simulink model "soc_pmsm_singlecpu_ref"  (R2023b)
settings: Solver=FixedStepAuto  StartTime=0.0  StopTime=1  RelTol=1e-3  EnableMultiTasking=on
InitFcn:
  | soc_mcb_pmsm_foc_sensorless_f28379d_data;
  | coeff = .007*Ts/50e-6;
model workspace (MAT data in the model file):
  mwTaskManagerKernelLatency = 0
values from neighbouring files (symbols this model uses):
  dataType = 'single'    [soc_mcb_pmsm_foc_sensorless_f28379d_data.m]
  inverter = mcb_SetInverterParameters('BoostXL-DRV8305')    [soc_mcb_pmsm_foc_sensorless_f28379d_data.m]
  PI_params = mcb.internal.SetControllerParameters(pmsm,inverter,PU_System,T_pwm,2*Ts,Ts_speed)    [soc_mcb_pmsm_foc_sensorless_f28379d_data.m]
  pmsm = mcb_SetPMSMMotorParameters('custom')    [soc_mcb_pmsm_foc_sensorless_f28379d_data.m]
  PU_System = mcb_SetPUSystem(pmsm,inverter)    [soc_mcb_pmsm_foc_sensorless_f28379d_data.m]
  Ts = T_pwm    (= 5e-05)    [soc_mcb_pmsm_foc_sensorless_f28379d_data.m]
  Ts_speed = 10*Ts    (= 0.0005)    [soc_mcb_pmsm_foc_sensorless_f28379d_data.m]
  Vd_Ref_openLoop_PU = Speed_openLoop_PU    (= 0.1)    [soc_mcb_pmsm_foc_sensorless_f28379d_data.m]
undefined symbols (not defined in the file or in its folder): soc_pmsm_singlecpu_ref
libraries: mcbcontrolslib x10, prociolib x5, simulink x4, slpidlib x3, mcbpositiondecoderlib x2
settings Model: ExtModeTrigDuration=8  Creator=The MathWorks, Inc.  LastModifiedBy=The MathWorks, Inc.
settings SolverCC: AlgebraicLoopSolver=TrustRegion  PositivePriorityOrder=on  MaxZcPerStep=1
settings DataIOCC: SaveOutput=off  DSMLogging=off
settings OptimizationCC: DefaultUnderspecifiedDataType=single  EnhancedBackFolding=on  PassReuseOutputArgsAs=Individual arguments  MaxStackSize=1024  OptimizeBlockOrder=speed  DifferentSizesBufferReuse=on  OptimizationCustomize=off  DenormalBehavior=FlushToZero  EfficientTunableParamExpr=on
settings DebuggingCC: IntegerOverflowMsg=none  ParameterPrecisionLossMsg=none  ParameterTunabilityLossMsg=error  UnconnectedInputMsg=warning  UnconnectedOutputMsg=warning  UnconnectedLineMsg=warning
settings HardwareCC: ProdBitPerChar=16  ProdBitPerInt=16  ProdBitPerPointer=32  ProdBitPerSizeT=32  ProdBitPerPtrDiffT=32  ProdLargestAtomicInteger=Integer  ProdLargestAtomicFloat=None  ProdWordSize=16  ProdLongLongMode=on  ProdHWDeviceType=Texas Instruments->C2000  HardwareBoardFeatureSet=SoCBlockset
settings ModelReferenceCC: EnableRefExpFcnMdlSchedulingChecks=on  ModelReferenceNumInstancesAllowed=Single
settings SFSimCC: MATLABDynamicMemAlloc=off
settings RTWCC: Description=Embedded Coder  SystemTargetFile=ert.tlc  HardwareBoard=TI Delfino F28379D LaunchPad  TLCOptions="-aInlineSetEventsForThisBaseRateFcn=TLC_FALSE -aSuppressMultiTaskScheduler=TLC_FALSE   -aRateBasedStepFcn=1"  TemplateMakefile=ert_default_tmf  Toolchain=Texas Instruments Code Composer Studio (C2000)  DLArmComputeVersion=19.05
settings CodeAppCC: ForceParamTrailComments=on  IgnoreCustomStorageClasses=off  MaxIdLength=64  OperatorAnnotations=on  SimulinkDataObjDesc=on  SFDataObjDesc=on  InsertBlockDesc=on
settings ERTTargetCC: CodeReplacementLibrary=TI C28x  ExtModeTransport=4  ExtModeStaticAlloc=on  ExtModeStaticAllocSize=10000  ExtModeMexFile=ext_xcp  ExtModeIntrfLevel=Level2 - Open

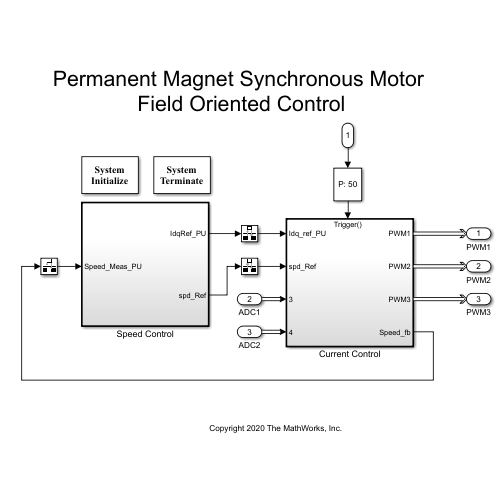
[thumbnail: Simulink's stored preview of the top-level diagram]
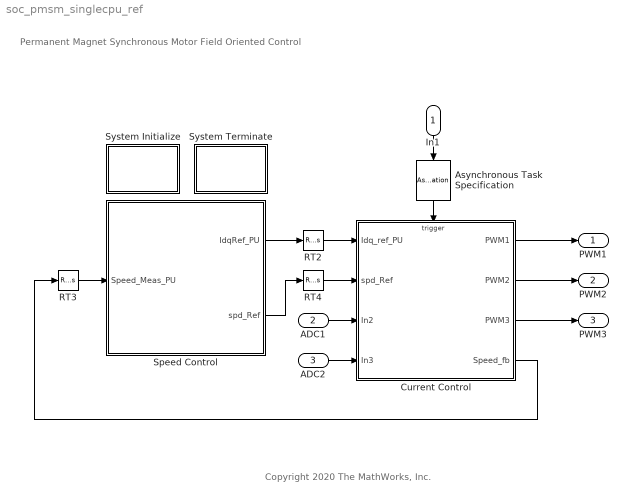
== system soc_pmsm_singlecpu_ref ==
  note: Permanent Magnet Synchronous Motor
      | Field Oriented Control
  note: Copyright 2020 The MathWorks, Inc.
  In1 : Inport  OutputFunctionCall=on
  ADC1 : Inport  OutputPortMessageModes=m  Port=2
  ADC2 : Inport  OutputPortMessageModes=m  Port=3
  Asynchronous Task Specification : AsynchronousTaskSpecification  TaskPriority=50
  Current Control : Subsystem
  RT2 : RateTransition  Deterministic=off
  RT3 : RateTransition  Deterministic=off  OutPortSampleTime=Ts_speed
  RT4 : RateTransition  Deterministic=off
  Speed Control : Subsystem  TreatAsAtomicUnit=on  SystemSampleTime=Ts_speed
  System Initialize : Subsystem  mask(System Initialize){ShowInLibBrowser=0}
      mask prompts: ShowInLibBrowser "Simulink:masks:CustCodeMaskParam1_MP"
      settings: CopyFcn=cccopyfcn(gcb)  OpenFcn=ccopenfcn('System Initialize Function')
      mask Help: eval('feval(''rtwprivate'',''rtwhelpview'',''rtw_sys_initialize_block'')');
      mask Display: disp('System\nInitialize');
  System Terminate : Subsystem  mask(System Terminate){ShowInLibBrowser=0}
      mask prompts: ShowInLibBrowser "Simulink:masks:CustCodeMaskParam1_MP"
      settings: CopyFcn=cccopyfcn(gcb)  OpenFcn=ccopenfcn('System Terminate Function')
      mask Help: eval('feval(''rtwprivate'',''rtwhelpview'',''rtw_sys_terminate_block'')');
      mask Display: disp('System\nTerminate');
  PWM1 : Outport  InputPortMessageModes=m
  PWM2 : Outport  InputPortMessageModes=m  Port=2
  PWM3 : Outport  InputPortMessageModes=m  Port=3
  wires:
  RT2/1 -> Current Control/1(Idq_ref_PU)
  ADC2/1 -> Current Control/4(In3)
  Current Control/4(Speed_fb) -> RT3/1
  ADC1/1 -> Current Control/3(In2)
  In1/1 -> Asynchronous Task Specification/1
  Current Control/2(PWM2) -> PWM2/1
  Current Control/1(PWM1) -> PWM1/1
  Current Control/3(PWM3) -> PWM3/1
  Speed Control/1(IdqRef_PU) -> RT2/1
  RT3/1 -> Speed Control/1(Speed_Meas_PU)
  RT4/1 -> Current Control/2(spd_Ref)
  Asynchronous Task Specification/1 -> Current Control/Trigger
  Speed Control/2(spd_Ref) -> RT4/1

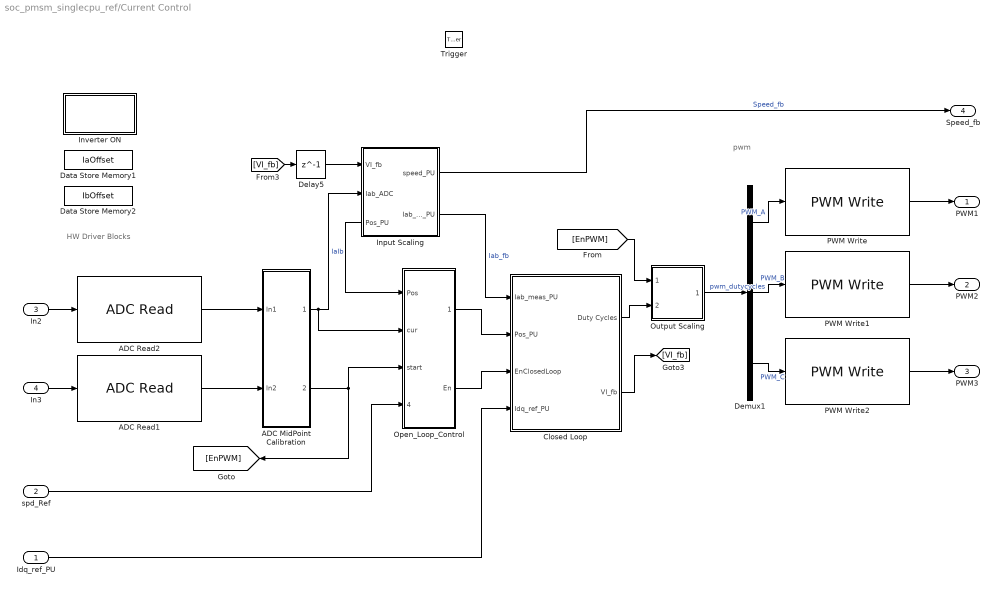
== system soc_pmsm_singlecpu_ref/Current Control ==
  note: pwm
  note: HW Driver Blocks
  Idq_ref_PU : Inport
  spd_Ref : Inport  Port=2
  In2 : Inport  Port=3
  In3 : Inport  Port=4
  Trigger : TriggerPort  TriggerType=function-call  VariantControl=Variant  PortDimensions=1
  ADC MidPoint Calibration : Subsystem
  ADC Read1 : prociolib/ADC Read  DataType=uint16  SampleTime=-1  NumCh=1  PeripheralConfigBtnCtrl=0  BlockSID=soc_pmsm_singlecpu_ref:512
  ADC Read2 : prociolib/ADC Read  DataType=uint16  SampleTime=-1  NumCh=1  PeripheralConfigBtnCtrl=0  BlockSID=soc_pmsm_singlecpu_ref:717
  Closed Loop : Subsystem
  Data Store Memory1 : DataStoreMemory  DataStoreName=IaOffset  ReadBeforeWriteMsg=warning  WriteAfterWriteMsg=warning  WriteAfterReadMsg=warning  InitialValue=inverter.CtSensAOffset  ShowAdditionalParam=off
  Data Store Memory2 : DataStoreMemory  DataStoreName=IbOffset  ReadBeforeWriteMsg=warning  WriteAfterWriteMsg=warning  WriteAfterReadMsg=warning  InitialValue=inverter.CtSensBOffset  ShowAdditionalParam=off
  Delay5 : Delay  DelayLength=1
  Demux1 : Demux  Outputs=3
  Input Scaling : Subsystem
      settings: PortSchema="{\"entries\":[{\"content\":{\"sides\":[{\"content\":{\"connectorIds\":[\"In1\",\"In2\",\"Out3\"]},\"type\":\"ConnectorPlacement.EquallySpacedRectSide\",\"uuid\":\"6d6167e7-0996-4b81-a35a-1346d5f5bdac\"},{\"content\":{\"connectorIds\":[\"Out1\",\"Out2\"],\"side\":\"RIGHT\"},\"type\":\"ConnectorPlacement.EquallySpacedRectSide\",\"uuid\":\"bac86f6f-215c-4b7d-8f06-4a6da7918799\"},{\"content\":{\"connectorIds\":[],\"side\":\"TOP\"},\"type\":\"ConnectorPlacement.EquallySpacedRectSide\",\"uuid\":\"65876525-48d1-40c6-98ca-4ecaae4f0bb2\"},{\"content\":{\"connectorIds\":[],\"side\":\"HIDDEN\"},\"type\":\"ConnectorPlacement.EquallySpacedRectSide\",\"uuid\":\"fe89acd2-2a3e-478b-951b-0712bf130e60\"}]},\"type\":\"ConnectorPlacement.EquallySpacedConnector\",\"uuid\":\"d7bb3362-92d6-4e3b-9b7c-91cd383782b7\"}],\"packageUris\":[\"http://schema.mathworks.com/mf0/Connector/R2020b\"],\"version\":\"1.0\"}"
  Inverter ON : Subsystem  mask(System Outputs){ShowInLibBrowser=0}
      mask prompts: ShowInLibBrowser "Simulink:masks:CustCodeMaskParam1_MP"
      settings: CopyFcn=cccopyfcn(gcb)  OpenFcn=ccopenfcn('System Outputs Function')
      mask Help: eval('feval(''rtwprivate'',''rtwhelpview'',''rtw_sys_outputs_block'')');
      mask Display: disp('System\nOutputs');
  Open_Loop_Control : Subsystem
  Output Scaling : Subsystem
  PWM Write : prociolib/PWM Write  ShowPeriodInp=off  ShowPhaseInp=off  PeripheralConfigBtnCtrl=0  BlockSID=soc_pmsm_singlecpu_ref:666
  PWM Write1 : prociolib/PWM Write  ShowPeriodInp=off  ShowPhaseInp=off  PeripheralConfigBtnCtrl=0  BlockSID=soc_pmsm_singlecpu_ref:667
  PWM Write2 : prociolib/PWM Write  ShowPeriodInp=off  ShowPhaseInp=off  PeripheralConfigBtnCtrl=0  BlockSID=soc_pmsm_singlecpu_ref:668
  PWM1 : Outport
  PWM2 : Outport  Port=2
  PWM3 : Outport  Port=3
  Speed_fb : Outport  Port=4  InitialOutput=0  VectorParamsAs1DForOutWhenUnconnected=off
  wires:
  Closed Loop/1(Duty Cycles) -> Output Scaling/2(Vabc_ref)
  Delay5/1 -> Input Scaling/1(VI_fb)
  Output Scaling/1(PWM_Duty_Cycles) -> Demux1/1  "pwm_dutycycles"
  Closed Loop/2(VI_fb) -> [VI_fb]
  PWM Write1/1 -> PWM2/1
  In3/1 -> ADC Read1/1
  Input Scaling/2(Iab_meas_PU) -> Closed Loop/1(Iab_meas_PU)  "Iab_fb"
  Input Scaling/1(speed_PU) -> Speed_fb/1  "Speed_fb"
  In2/1 -> ADC Read2/1
  [VI_fb] -> Delay5/1
  ADC Read2/1 -> ADC MidPoint Calibration/1(In1)
  Idq_ref_PU/1 -> Closed Loop/4(Idq_ref_PU)
  ADC Read1/1 -> ADC MidPoint Calibration/2(In2)
  PWM Write2/1 -> PWM3/1
  PWM Write/1 -> PWM1/1
  Demux1/3 -> PWM Write2/1  "PWM_C"
  Demux1/2 -> PWM Write1/1  "PWM_B"
  Demux1/1 -> PWM Write/1  "PWM_A"
  ADC MidPoint Calibration/1(Iab_ADC) -> Open_Loop_Control/2(cur), Input Scaling/2(Iab_ADC)  "IaIb"
  spd_Ref/1 -> Open_Loop_Control/4(spd_Ref)
  Open_Loop_Control/1(Pos_PU) -> Closed Loop/2(Pos_PU)
  Open_Loop_Control/2(En) -> Closed Loop/3(EnClosedLoop)
  ADC MidPoint Calibration/2(EnPWM) -> [EnPWM], Open_Loop_Control/3(start)
  [EnPWM] -> Output Scaling/1(EnPWM)
  Input Scaling/3(Pos_PU) -> Open_Loop_Control/1(Pos)

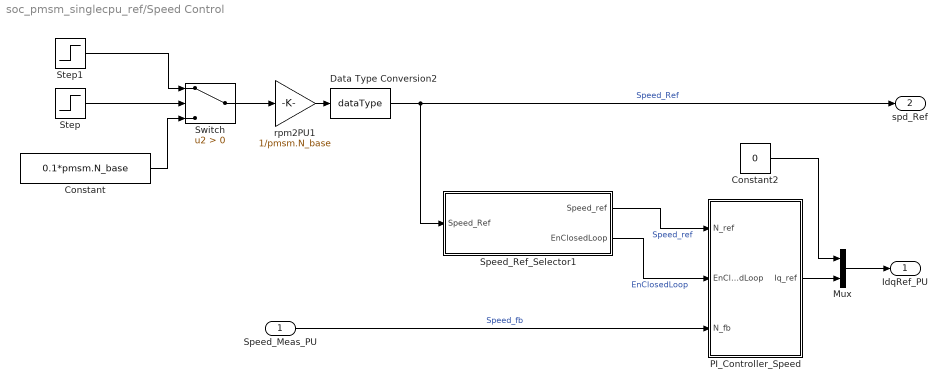
== system soc_pmsm_singlecpu_ref/Speed Control ==
  Speed_Meas_PU : Inport
  Constant : Constant  Value=0.1*pmsm.N_base  SampleTime=-1
  Constant2 : Constant  Value=0  OutDataTypeStr=dataType
  Data Type Conversion2 : DataTypeConversion  OutDataTypeStr=dataType  RndMeth=Simplest  SaturateOnIntegerOverflow=off
  Mux : Mux  Inputs=2
  PI_Controller_Speed : Subsystem
  Speed_Ref_Selector1 : Subsystem
  Step : Step  Time=.05
  Step1 : Step  Time=.3  Before=0.5*pmsm.N_base  After=0.7*pmsm.N_base
  Switch : Switch  Criteria=u2 > Threshold  SaturateOnIntegerOverflow=off  InputSameDT=off
  rpm2PU1 : Gain  Gain=1/pmsm.N_base  RndMeth=Simplest  OutDataTypeStr=Inherit: Same as input
  IdqRef_PU : Outport  VectorParamsAs1DForOutWhenUnconnected=off
  spd_Ref : Outport  Port=2  VectorParamsAs1DForOutWhenUnconnected=off
  wires:
  Speed_Meas_PU/1 -> PI_Controller_Speed/3(N_fb)  "Speed_fb"
  Mux/1 -> IdqRef_PU/1
  Constant2/1 -> Mux/1
  PI_Controller_Speed/1(Iq_ref) -> Mux/2
  Data Type Conversion2/1 -> Speed_Ref_Selector1/1(Speed_Ref), spd_Ref/1  "Speed_Ref"
  rpm2PU1/1 -> Data Type Conversion2/1
  Speed_Ref_Selector1/1(Speed_ref) -> PI_Controller_Speed/1(N_ref)  "Speed_ref"
  Speed_Ref_Selector1/2(EnClosedLoop) -> PI_Controller_Speed/2(EnClosedLoop)  "EnClosedLoop"
  Constant/1 -> Switch/3
  Step/1 -> Switch/2
  Step1/1 -> Switch/1
  Switch/1 -> rpm2PU1/1

== system soc_pmsm_singlecpu_ref/System Initialize ==

== system soc_pmsm_singlecpu_ref/System Terminate ==

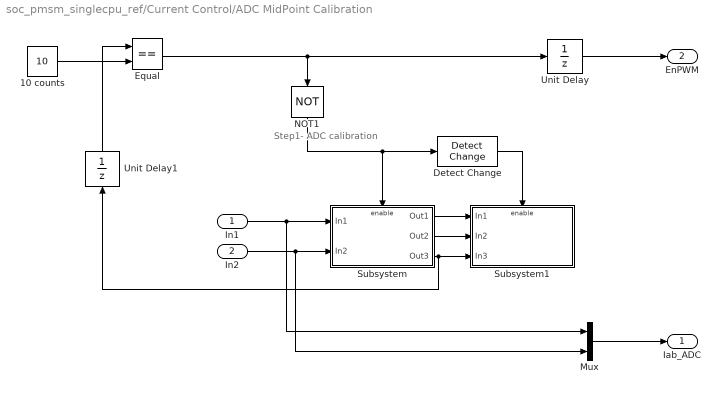
== system soc_pmsm_singlecpu_ref/Current Control/ADC MidPoint Calibration ==
  note: Step1- ADC calibration
  In1 : Inport
  In2 : Inport  Port=2
  10 counts : Constant  Value=10
  Detect Change : simulink/Logic and Bit Operations/Detect Change  vinit=1  OutDataTypeStr=boolean
  Equal : RelationalOperator  Operator===  OutDataTypeStr=boolean  RndMeth=Simplest  InputSameDT=off
  Mux : Mux  Inputs=2
  NOT1 : Logic  Operator=NOT  IconShape=distinctive  AllPortsSameDT=off  OutDataTypeStr=boolean
  Subsystem : Subsystem
  Subsystem1 : Subsystem
  Unit Delay : UnitDelay  SampleTime=-1  HasFrameUpgradeWarning=on
  Unit Delay1 : UnitDelay  SampleTime=-1  HasFrameUpgradeWarning=on
  Iab_ADC : Outport
  EnPWM : Outport  Port=2
  wires:
  Equal/1 -> NOT1/1, Unit Delay/1
  Subsystem/1(Out1) -> Subsystem1/1(In1)
  Detect Change/1 -> Subsystem1/Enable
  Subsystem/3(Out3) -> Unit Delay1/1, Subsystem1/3(In3)
  Subsystem/2(Out2) -> Subsystem1/2(In2)
  In1/1 -> Mux/1, Subsystem/1(In1)
  In2/1 -> Mux/2, Subsystem/2(In2)
  Mux/1 -> Iab_ADC/1
  Unit Delay/1 -> EnPWM/1
  NOT1/1 -> Subsystem/Enable, Detect Change/1
  Unit Delay1/1 -> Equal/1
  10 counts/1 -> Equal/2

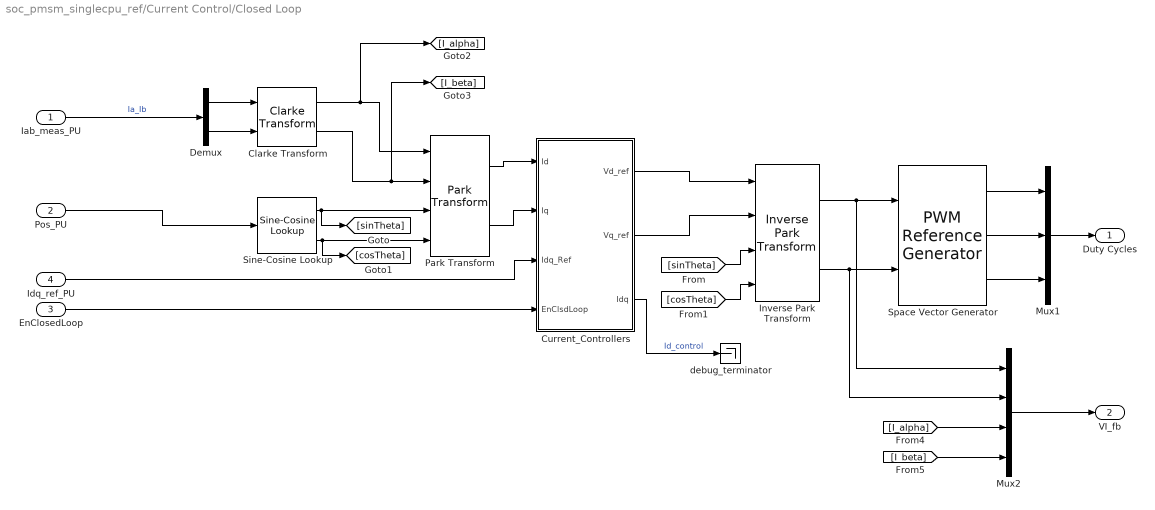
== system soc_pmsm_singlecpu_ref/Current Control/Closed Loop ==
  Iab_meas_PU : Inport
  Pos_PU : Inport  Port=2
  EnClosedLoop : Inport  Port=3
  Idq_ref_PU : Inport  Port=4
  Clarke Transform : mcbcontrolslib/Clarke Transform  VariantControl=Variant2  PhaseInput=Two inputs  EnPowerInv=off
  Current_Controllers : Subsystem
  Demux : Demux  Outputs=2
  Inverse Park Transform : mcbcontrolslib/Inverse Park Transform  PhaseInput=Two inputs  AxisAlignment=D-axis  ThetaInput=Sine and Cosine electrical position  AngleInput=Per-unit  N_points=1024
  Mux1 : Mux  Inputs=3
  Mux2 : Mux
  Park Transform : mcbcontrolslib/Park Transform  PhaseInput=Two inputs  AxisAlignment=D-axis  ThetaInput=Sine and Cosine electrical position  AngleInput=Per-unit  N_points=1024
  Sine-Cosine Lookup : mcbcontrolslib/Sine-Cosine Lookup  AngleInput=Per-unit  N_points=1024
  Space Vector Generator : mcbcontrolslib/PWM Reference Generator  inSignal=Valphabeta  modType=SVM: space vector modulation
  debug_terminator : Terminator
  Duty Cycles : Outport  VectorParamsAs1DForOutWhenUnconnected=off
  VI_fb : Outport  Port=2  VectorParamsAs1DForOutWhenUnconnected=off
  wires:
  Current_Controllers/1(Vd_ref) -> Inverse Park Transform/1
  [cosTheta] -> Inverse Park Transform/4
  [I_beta] -> Mux2/4
  Inverse Park Transform/2 -> Space Vector Generator/2, Mux2/2
  Inverse Park Transform/1 -> Space Vector Generator/1, Mux2/1
  [sinTheta] -> Inverse Park Transform/3
  Mux2/1 -> VI_fb/1
  Clarke Transform/1 -> [I_alpha], Park Transform/1
  Current_Controllers/2(Vq_ref) -> Inverse Park Transform/2
  Clarke Transform/2 -> [I_beta], Park Transform/2
  Sine-Cosine Lookup/1 -> [sinTheta], Park Transform/3
  [I_alpha] -> Mux2/3
  Space Vector Generator/1 -> Mux1/1
  Space Vector Generator/3 -> Mux1/3
  Mux1/1 -> Duty Cycles/1
  Sine-Cosine Lookup/2 -> Park Transform/4, [cosTheta]
  Space Vector Generator/2 -> Mux1/2
  Park Transform/1 -> Current_Controllers/1(Id)
  Park Transform/2 -> Current_Controllers/2(Iq)
  Demux/1 -> Clarke Transform/1
  Demux/2 -> Clarke Transform/2
  Iab_meas_PU/1 -> Demux/1  "Ia_Ib"
  Idq_ref_PU/1 -> Current_Controllers/3(Idq_Ref)
  Current_Controllers/3(Idq) -> debug_terminator/1  "Id_control"
  Pos_PU/1 -> Sine-Cosine Lookup/1
  EnClosedLoop/1 -> Current_Controllers/4(EnClsdLoop)

== system soc_pmsm_singlecpu_ref/Current Control/Input Scaling ==
  note: This filter is required to correct DC offset,
      | which helps to estimate position more accurately.
  note: Current Measurements
  note: Position & Speed Measurements
  VI_fb : Inport
  Iab_ADC : Inport  Port=2
  Calculate Phase Currents : Subsystem
  Calculate position and speed : Subsystem
  High pass filter : Subsystem
  speed_PU : Outport
  Iab_meas_PU : Outport  Port=2
  Pos_PU : Outport  Port=3
  wires:
  Calculate Phase Currents/1(Iab_meas_PU) -> Iab_meas_PU/1
  Iab_ADC/1 -> Calculate Phase Currents/1(Iab_ADC)
  VI_fb/1 -> High pass filter/1(In1)
  Calculate position and speed/2(Pos_PU) -> Pos_PU/1
  Calculate position and speed/1(speed_PU) -> speed_PU/1
  High pass filter/1(Out1) -> Calculate position and speed/1(VI_fb)

== system soc_pmsm_singlecpu_ref/Current Control/Inverter ON ==

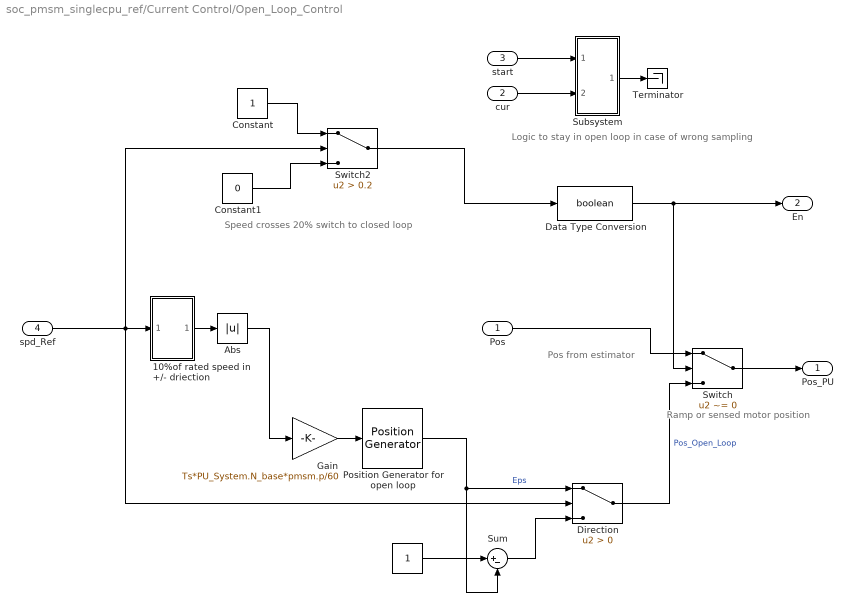
== system soc_pmsm_singlecpu_ref/Current Control/Open_Loop_Control ==
  note: Logic to stay in open loop in case of wrong sampling
  note: Speed crosses 20% switch to closed loop
  note: Pos from estimator
  note: Ramp or sensed motor position
  Pos : Inport
  cur : Inport  Port=2
  start : Inport  Port=3
  spd_Ref : Inport  Port=4
  " " : Constant  OutDataTypeStr=dataType  SampleTime=-1
  10%of rated speed in +/- driection : Subsystem
  Abs : Abs  SaturateOnIntegerOverflow=off
  Constant : Constant  OutDataTypeStr=uint16
  Constant1 : Constant  Value=0  OutDataTypeStr=uint16
  Data Type Conversion : DataTypeConversion  OutDataTypeStr=boolean  RndMeth=Simplest  SaturateOnIntegerOverflow=off
  Direction : Switch  Criteria=u2 > Threshold  OutDataTypeStr=dataType  RndMeth=Simplest  SaturateOnIntegerOverflow=off  InputSameDT=off
  Gain : Gain  Gain=Ts*PU_System.N_base*pmsm.p/60  OutDataTypeStr=Inherit: Same as input  ParamDataTypeStr=Inherit: Same as input
  Position Generator for open loop : mcbcontrolslib/Position Generator  AngleOutput=Per-unit  ExternalReset=none  Offset=0
  Subsystem : Subsystem
  Sum : Sum  Inputs=|+-  RndMeth=Simplest  OutDataTypeStr=Inherit: Same as first input
  Switch : Switch  Criteria=u2 ~= 0  Threshold=0.1  SaturateOnIntegerOverflow=off  InputSameDT=off
  Switch2 : Switch  Criteria=u2 > Threshold  Threshold=0.2  SaturateOnIntegerOverflow=off  InputSameDT=off
  Terminator : Terminator
  Pos_PU : Outport
  En : Outport  Port=2
  wires:
  Constant1/1 -> Switch2/3
  Constant/1 -> Switch2/1
  Pos/1 -> Switch/1
  Switch/1 -> Pos_PU/1
  Gain/1 -> Position Generator for open loop/1
  Switch2/1 -> Data Type Conversion/1
  spd_Ref/1 -> Switch2/2, Direction/2, 10%of rated speed in +/- driection/1(In1)
  Sum/1 -> Direction/3
  " "/1 -> Sum/1
  Position Generator for open loop/1 -> Direction/1, Sum/2  "Eps"
  Direction/1 -> Switch/3  "Pos_Open_Loop"
  Abs/1 -> Gain/1
  10%of rated speed in +/- driection/1(Out1) -> Abs/1
  cur/1 -> Subsystem/2(In1)
  start/1 -> Subsystem/1(start)
  Data Type Conversion/1 -> En/1, Switch/2
  Subsystem/1(Close) -> Terminator/1

== system soc_pmsm_singlecpu_ref/Current Control/Output Scaling ==
  EnPWM : Inport
  Vabc_ref : Inport  Port=2
  Constant : Constant  Value=0.5  OutDataTypeStr=dataType  SampleTime=-1
  Constant1 : Constant  Value=0  OutDataTypeStr=single
  Mux : Mux  Inputs=3
  One_by_Two : Gain  Gain=0.5  RndMeth=Simplest  OutDataTypeStr=Inherit: Same as input
  Sum : Sum  Inputs=|++
  Switch : Switch  Criteria=u2 > Threshold  SaturateOnIntegerOverflow=off  InputSameDT=off
  PWM_Duty_Cycles : Outport
  wires:
  Constant/1 -> Sum/2
  Vabc_ref/1 -> One_by_Two/1
  One_by_Two/1 -> Sum/1
  Mux/1 -> Switch/3
  Constant1/1 -> Mux/3, Mux/1, Mux/2
  Sum/1 -> Switch/1  "PWM_Duty_Cycles"
  EnPWM/1 -> Switch/2
  Switch/1 -> PWM_Duty_Cycles/1  "pwm_dutycycles"

== system soc_pmsm_singlecpu_ref/Speed Control/PI_Controller_Speed ==
  N_ref : Inport
  EnClosedLoop : Inport  Port=2
  N_fb : Inport  Port=3
  Discrete PI Controller with anti-windup & reset : slpidlib/PID Controller  Controller=PI  Form=Parallel  TimeDomain=Discrete-time  UseExternalTs=off  SampleTime=-1  IntegratorMethod=Forward Euler  FilterMethod=Forward Euler  ControllerParametersSource=external  P=1  I=1  UseKiTs=on  D=0  N=100  UseFilter=on  TunerSelectOption=Transfer Function Based (PID Tuner App)  InitialConditionSource=external  InitialConditionForIntegrator=0  InitialConditionForFilter=0  DifferentiatorICPrevScaledInput=0  ExternalReset=level  TrackingMode=off  Kt=1  LimitOutput=on  SatLimitsSource=internal  UpperSaturationLimit=1  LowerSaturationLimit=-1  LinearizeAsGain=on  AntiWindupMode=clamping  Kb=1  LimitIntegrator=off  UpperIntegratorSaturationLimit=inf  LowerIntegratorSaturationLimit=-inf  RndMeth=Simplest  POutMin=[]  POutMax=[]  IOutMin=[]  IOutMax=[]  DOutMin=[]  DOutMax=[]  NOutMin=[]  NOutMax=[]  SumOutMin=[]  SumOutMax=[]  SaturationOutDataTypeStr=Inherit: Inherit via back propagation  SaturationOutMin=[]  SaturationOutMax=[]  PParamMin=[]  PParamMax=[]  IParamMin=[]  IParamMax=[]  DParamMin=[]  DParamMax=[]  NParamMin=[]  NParamMax=[]  KbParamMin=[]  KbParamMax=[]  KtParamMin=[]  KtParamMax=[]  KbOutMin=[]  KbOutMax=[]  KtOutMin=[]  KtOutMax=[]  IntegratorOutMin=[]  IntegratorOutMax=[]  FilterOutMin=[]  FilterOutMax=[]  SumI1OutMin=[]  SumI1OutMax=[]  SumI2OutMin=[]  SumI2OutMax=[]  SumI3OutMin=[]  SumI3OutMax=[]  SumI4OutMin=[]  SumI4OutMax=[]  SumDOutMin=[]  SumDOutMax=[]  DifferentiatorOutMin=[]  DifferentiatorOutMax=[]  FilterDiffOutCoefMin=[]  FilterDiffOutCoefMax=[]  ReciprocalOutMin=[]  ReciprocalOutMax=[]  SumDenOutMin=[]  SumDenOutMax=[]  SumNumOutMin=[]  SumNumOutMax=[]  DivideOutMin=[]  DivideOutMax=[]  UdiffTsProdOutMin=[]  UdiffTsProdOutMax=[]  NTsProdOutMin=[]  NTsProdOutMax=[]  UintegralTsProdOutMin=[]  UintegralTsProdOutMax=[]  UngainTsProdOutMin=[]  UngainTsProdOutMax=[]  ClampingZeroOutDataTypeStr=Inherit: Inherit via back propagation  ClampingZeroOutMin=[]  ClampingZeroOutMax=[]  FilterDenConstantOutDataTypeStr=Inherit: Inherit via back propagation  FilterDenConstantOutMin=[]  FilterDenConstantOutMax=[]  PCopyOutDataTypeStr=Inherit: Inherit via back propagation  PCopyOutMin=[]  PCopyOutMax=[]  NCopyOutDataTypeStr=Inherit: Inherit via back propagation  NCopyOutMin=[]  NCopyOutMax=[]  IntegratorContinuousStateAttributes=''  IntegratorStateMustResolveToSignalObject=off  IntegratorRTWStateStorageClass=Auto  FilterContinuousStateAttributes=''  FilterStateMustResolveToSignalObject=off  FilterRTWStateStorageClass=Auto  ParallelPVariant=ExternalParameters  IdealPVariant=Disabled  IVariant=ExternalParameters  DVariant=Disabled  IntegratorVariant=Discrete  SatVariant=Enabled  AWVariant=DiscClampingParallel  PCopyVariant=Disabled  TRVariant=Disabled  FdbkBlocksVariant=Forward  IdealPFdbkVariant=Disabled  SatFdbkVariant=Disabled  DerivativeFilterVariant=Disabled  NVariant=Disabled  NCopyVariant=Disabled_SignalSpec  FilterICVariant=Disabled  IntegratorICVariant=ExternalICs  ExternalResetVariant=ExternalReset  TRSumVariant=Passthrough  SumFdbkVariant=Disabled  SumVariant=Sum_PI  TsampFilterVariant=InternalTs  TsampNgainVariant=Passthrough  TsampIntegralVariant=Disabled_SignalSpec  ExternalSaturationOutDataTypeStr=Inherit: Same as second input
      settings: LibrarySourceBlock=mcbcontrolslib/PI Controller
  Ki1 : Constant  Value=PI_params.Ki_speed*Ts_speed  OutDataTypeStr=dataType  SampleTime=-1
  Ki2 : Constant  Value=0  OutDataTypeStr=dataType  SampleTime=-1
  Kp1 : Constant  Value=PI_params.Kp_speed  OutDataTypeStr=dataType  SampleTime=-1
  Logical Operator : Logic  Operator=NOT  IconShape=distinctive  AllPortsSameDT=off  OutDataTypeStr=boolean
  Sum : Sum  Inputs=|+-  OutDataTypeStr=Inherit: Same as first input
  Iq_ref : Outport  VectorParamsAs1DForOutWhenUnconnected=off
  wires:
  Discrete PI Controller with anti-windup & reset/1 -> Iq_ref/1
  Ki1/1 -> Discrete PI Controller with anti-windup & reset/3
  Kp1/1 -> Discrete PI Controller with anti-windup & reset/2
  N_fb/1 -> Sum/2
  N_ref/1 -> Sum/1
  Sum/1 -> Discrete PI Controller with anti-windup & reset/1
  Logical Operator/1 -> Discrete PI Controller with anti-windup & reset/4
  Ki2/1 -> Discrete PI Controller with anti-windup & reset/5
  EnClosedLoop/1 -> Logical Operator/1

== system soc_pmsm_singlecpu_ref/Speed Control/Speed_Ref_Selector1 ==
  note: En Closed loop
  Speed_Ref : Inport
  Ki3 : Constant  Value=0  OutDataTypeStr=dataType  SampleTime=-1
  Ki4 : Constant  OutDataTypeStr=dataType  SampleTime=-1
  Switch2 : Switch  Criteria=u2 > Threshold  Threshold=.2  SaturateOnIntegerOverflow=off  InputSameDT=off
  Unit Delay : UnitDelay  SampleTime=-1  HasFrameUpgradeWarning=on
  Zero_Cancellation : mcbcontrolslib/IIR Filter  VariantControl=Low Pass Filter  VariantSelect=Low-pass  Filter_constant=.01*(Ts_speed/Ts)  advancedSettings=off  Ts=50e-6  cutOff_freq=1
  Speed_ref : Outport
  EnClosedLoop : Outport  Port=2
  wires:
  Speed_Ref/1 -> Unit Delay/1, Zero_Cancellation/1
  Switch2/1 -> EnClosedLoop/1
  Ki3/1 -> Switch2/3
  Ki4/1 -> Switch2/1
  Unit Delay/1 -> Switch2/2
  Zero_Cancellation/1 -> Speed_ref/1

== system soc_pmsm_singlecpu_ref/Current Control/ADC MidPoint Calibration/Subsystem ==
  In1 : Inport
  In2 : Inport  Port=2
  Enable : EnablePort
  Counter Free-Running : simulink/Sources/Counter Free-Running  NumBits=16  tsamp=-1
  Memory : Memory  InheritSampleTime=on
  Memory1 : Memory  InheritSampleTime=on
  Sum : Sum
  Sum1 : Sum
  Out1 : Outport  InitialOutput=2048
  Out2 : Outport  Port=2  InitialOutput=2048
  Out3 : Outport  Port=3  InitialOutput=2048
  wires:
  In1/1 -> Sum/1
  Memory/1 -> Sum/2
  Memory1/1 -> Sum1/2
  Sum/1 -> Memory/1, Out1/1
  In2/1 -> Sum1/1
  Sum1/1 -> Memory1/1, Out2/1
  Counter Free-Running/1 -> Out3/1

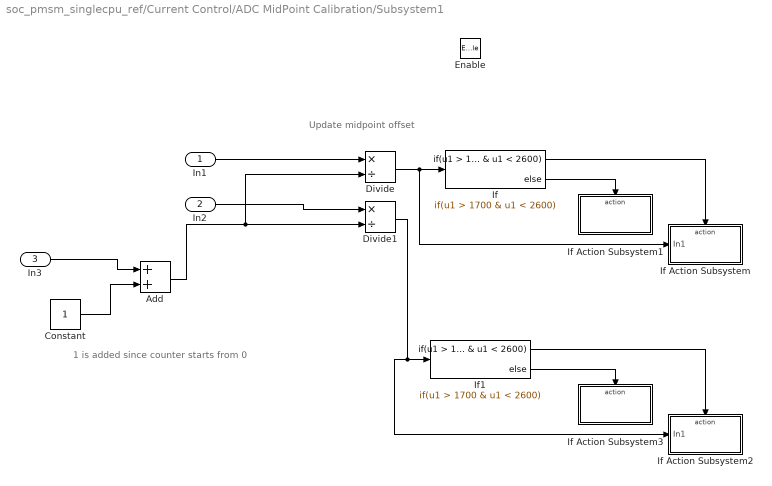
== system soc_pmsm_singlecpu_ref/Current Control/ADC MidPoint Calibration/Subsystem1 ==
  note: 1 is added since counter starts from 0
  note: Update midpoint offset
  In1 : Inport
  In2 : Inport  Port=2
  In3 : Inport  Port=3
  Enable : EnablePort
  Add : Sum
  Constant : Constant  SampleTime=-1
  Divide : Product  Inputs=*/  OutDataTypeStr=uint16
  Divide1 : Product  Inputs=*/  OutDataTypeStr=uint16
  If : If  IfExpression=u1 > 1700 & u1 < 2600
  If Action Subsystem : Subsystem  TreatAsAtomicUnit=on
  If Action Subsystem1 : Subsystem  TreatAsAtomicUnit=on
  If Action Subsystem2 : Subsystem  TreatAsAtomicUnit=on
  If Action Subsystem3 : Subsystem  TreatAsAtomicUnit=on
  If1 : If  IfExpression=u1 > 1700 & u1 < 2600
  wires:
  In1/1 -> Divide/1
  If1/2 -> If Action Subsystem3/Action
  In2/1 -> Divide1/1
  If1/1 -> If Action Subsystem2/Action
  Divide1/1 -> If Action Subsystem2/1(In1), If1/1
  If/1 -> If Action Subsystem/Action
  Add/1 -> Divide/2, Divide1/2
  If/2 -> If Action Subsystem1/Action
  Divide/1 -> If Action Subsystem/1(In1), If/1
  In3/1 -> Add/1
  Constant/1 -> Add/2

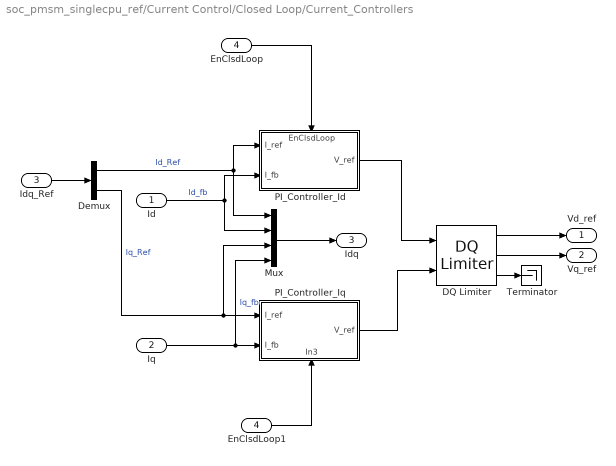
== system soc_pmsm_singlecpu_ref/Current Control/Closed Loop/Current_Controllers ==
  Id : Inport
  Iq : Inport  Port=2
  Idq_Ref : Inport  Port=3
  EnClsdLoop : Inport  Port=4
  DQ Limiter : mcbcontrolslib/DQ Limiter  satMethodInputType=Specify via dialog  satMethodSelected=D-Q equivalence  satLimitInputType=Specify via dialog  Vmax=0.95
  Demux : Demux  Outputs=2
  EnClsdLoop1 : InportShadow  Port=4
  Mux : Mux
  PI_Controller_Id : Subsystem
      settings: PortSchema="{\"entries\":[{\"content\":{\"sides\":[{\"content\":{\"connectorIds\":[\"In1\",\"In2\"]},\"type\":\"ConnectorPlacement.EquallySpacedRectSide\",\"uuid\":\"1dbe4538-5262-4de9-8cd0-6fe9721117d9\"},{\"content\":{\"connectorIds\":[\"Out1\"],\"side\":\"RIGHT\"},\"type\":\"ConnectorPlacement.EquallySpacedRectSide\",\"uuid\":\"73929c6b-82a2-4171-bcf4-852047833ed6\"},{\"content\":{\"connectorIds\":[\"In3\"],\"side\":\"TOP\"},\"type\":\"ConnectorPlacement.EquallySpacedRectSide\",\"uuid\":\"d145dc66-6457-4965-9d28-ee054dd23661\"},{\"content\":{\"connectorIds\":[],\"side\":\"HIDDEN\"},\"type\":\"ConnectorPlacement.EquallySpacedRectSide\",\"uuid\":\"26db549f-462f-46ef-aaa7-ab739cada5d6\"}]},\"type\":\"ConnectorPlacement.EquallySpacedConnector\",\"uuid\":\"507f0757-a119-4143-8cba-4226e39989e3\"}],\"packageUris\":[\"http://schema.mathworks.com/mf0/Connector/R2020b\"],\"version\":\"1.0\"}"
  PI_Controller_Iq : Subsystem
      settings: PortSchema="{\"entries\":[{\"content\":{\"sides\":[{\"content\":{\"connectorIds\":[\"In1\",\"In2\"]},\"type\":\"ConnectorPlacement.EquallySpacedRectSide\",\"uuid\":\"1dbe4538-5262-4de9-8cd0-6fe9721117d9\"},{\"content\":{\"connectorIds\":[\"Out1\"],\"side\":\"RIGHT\"},\"type\":\"ConnectorPlacement.EquallySpacedRectSide\",\"uuid\":\"73929c6b-82a2-4171-bcf4-852047833ed6\"},{\"content\":{\"connectorIds\":[],\"side\":\"TOP\"},\"type\":\"ConnectorPlacement.EquallySpacedRectSide\",\"uuid\":\"d145dc66-6457-4965-9d28-ee054dd23661\"},{\"content\":{\"connectorIds\":[\"In3\"],\"side\":\"BOTTOM\"},\"type\":\"ConnectorPlacement.EquallySpacedRectSide\",\"uuid\":\"758abaee-43c6-4dc5-aebc-88543f7390b7\"},{\"content\":{\"connectorIds\":[],\"side\":\"HIDDEN\"},\"type\":\"ConnectorPlacement.EquallySpacedRectSide\",\"uuid\":\"26db549f-462f-46ef-aaa7-ab739cada5d6\"}]},\"type\":\"ConnectorPlacement.EquallySpacedConnector\",\"uuid\":\"507f0757-a119-4143-8cba-4226e39989e3\"}],\"packageUris\":[\"http://schema.mathworks.com/mf0/Connector/R2020b\"],\"version\":\"1.0\"}"
  Terminator : Terminator
  Vd_ref : Outport  VectorParamsAs1DForOutWhenUnconnected=off
  Vq_ref : Outport  Port=2  VectorParamsAs1DForOutWhenUnconnected=off
  Idq : Outport  Port=3  VectorParamsAs1DForOutWhenUnconnected=off
  wires:
  Iq/1 -> Mux/4, PI_Controller_Iq/2(I_fb)  "Iq_fb"
  PI_Controller_Id/1(V_ref) -> DQ Limiter/1
  Id/1 -> PI_Controller_Id/2(I_fb), Mux/2  "Id_fb"
  Demux/1 -> PI_Controller_Id/1(I_ref), Mux/1  "Id_Ref"
  Demux/2 -> Mux/3, PI_Controller_Iq/1(I_ref)  "Iq_Ref"
  DQ Limiter/1 -> Vd_ref/1
  DQ Limiter/2 -> Vq_ref/1
  PI_Controller_Iq/1(V_ref) -> DQ Limiter/2
  DQ Limiter/3 -> Terminator/1
  Idq_Ref/1 -> Demux/1
  Mux/1 -> Idq/1
  EnClsdLoop/1 -> PI_Controller_Id/3(EnClsdLoop)
  EnClsdLoop1/1 -> PI_Controller_Iq/3(In3)

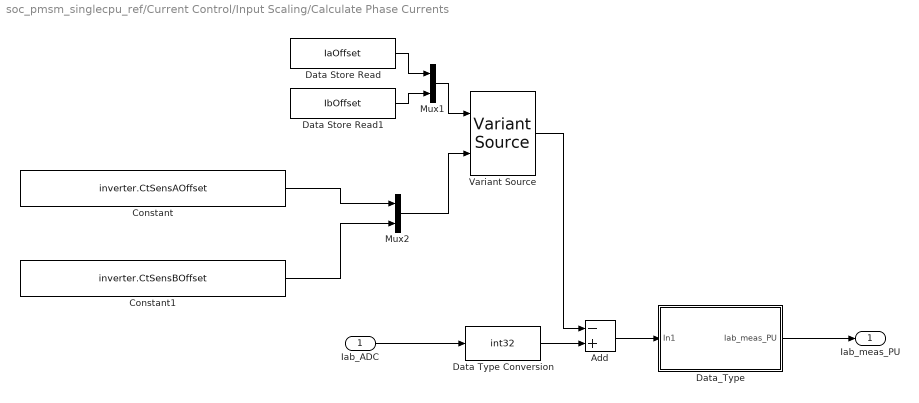
== system soc_pmsm_singlecpu_ref/Current Control/Input Scaling/Calculate Phase Currents ==
  Iab_ADC : Inport
  Add : Sum  Inputs=-+
  Constant : Constant  Value=inverter.CtSensAOffset  OutDataTypeStr=uint16  SampleTime=-1
  Constant1 : Constant  Value=inverter.CtSensBOffset  OutDataTypeStr=uint16  SampleTime=-1
  Data Store Read : DataStoreRead  DataStoreName=IaOffset  IndexOptions=Index vector (dialog)  Indices=1  OutputSizes=1
  Data Store Read1 : DataStoreRead  DataStoreName=IbOffset  IndexOptions=Index vector (dialog)  Indices=1  OutputSizes=1
  Data Type Conversion : DataTypeConversion  OutDataTypeStr=int32  ConvertRealWorld=Stored Integer (SI)  RndMeth=Simplest  SaturateOnIntegerOverflow=off
  Data_Type : Subsystem  Variant=on
  Mux1 : Mux  Inputs=2
  Mux2 : Mux  Inputs=2
  Variant Source : VariantSource  VariantControlMode=sim codegen switching  ShowConditionOnBlock=on
  Iab_meas_PU : Outport  VectorParamsAs1DForOutWhenUnconnected=off
  wires:
  Data Type Conversion/1 -> Add/2
  Add/1 -> Data_Type/1(In1)
  Data_Type/1(Iab_meas_PU) -> Iab_meas_PU/1
  Iab_ADC/1 -> Data Type Conversion/1
  Constant1/1 -> Mux2/2
  Constant/1 -> Mux2/1
  Mux2/1 -> Variant Source/2
  Data Store Read/1 -> Mux1/1
  Data Store Read1/1 -> Mux1/2
  Mux1/1 -> Variant Source/1
  Variant Source/1 -> Add/1

== system soc_pmsm_singlecpu_ref/Current Control/Input Scaling/Calculate position and speed ==
  VI_fb : Inport
  Demux : Demux  Outputs=2
  Flux Observer : Subsystem
  speed_PU : Outport
  Pos_PU : Outport  Port=2
  wires:
  VI_fb/1 -> Flux Observer/1(InputSignals)
  Demux/1 -> Pos_PU/1
  Demux/2 -> speed_PU/1
  Flux Observer/1(Position/Speed) -> Demux/1

== system soc_pmsm_singlecpu_ref/Current Control/Input Scaling/High pass filter ==
  In1 : Inport
  IIR Filter4 : mcbcontrolslib/IIR Filter  VariantControl=Low Pass Filter  VariantSelect=Low-pass  Filter_constant=coeff  advancedSettings=off  Ts=50e-6  cutOff_freq=1
  Sum : Sum  Inputs=|+-  RndMeth=Simplest
  Out1 : Outport
  wires:
  IIR Filter4/1 -> Sum/2
  In1/1 -> Sum/1, IIR Filter4/1
  Sum/1 -> Out1/1

== system soc_pmsm_singlecpu_ref/Current Control/Open_Loop_Control/10%of rated speed in +//- driection ==
  In1 : Inport
  Constant2 : Constant  Value=0.1  OutDataTypeStr=dataType
  Constant3 : Constant  Value=-0.1  OutDataTypeStr=dataType
  Switch1 : Switch  Criteria=u2 > Threshold  SaturateOnIntegerOverflow=off  InputSameDT=off
  Out1 : Outport
  wires:
  In1/1 -> Switch1/2
  Constant2/1 -> Switch1/1
  Constant3/1 -> Switch1/3
  Switch1/1 -> Out1/1

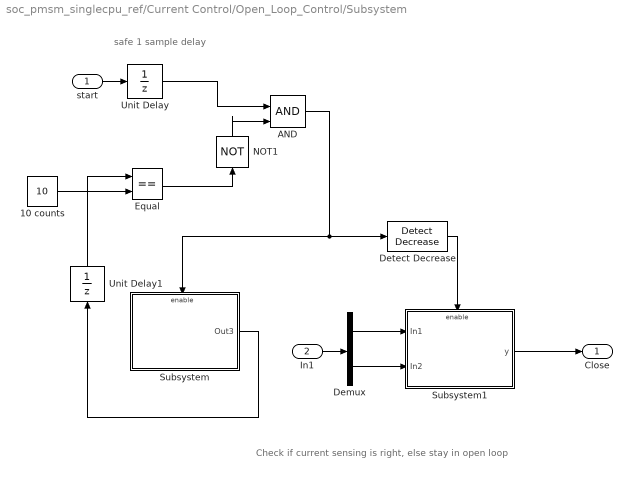
== system soc_pmsm_singlecpu_ref/Current Control/Open_Loop_Control/Subsystem ==
  note: safe 1 sample delay
  note: Check if current sensing is right, else stay in open loop
  start : Inport
  In1 : Inport  Port=2
  10 counts : Constant  Value=10
  AND : Logic  IconShape=distinctive  AllPortsSameDT=off  OutDataTypeStr=boolean
  Demux : Demux  Outputs=2
  Detect Decrease : simulink/Logic and Bit Operations/Detect Decrease  vinit=0.0  OutDataTypeStr=boolean
  Equal : RelationalOperator  Operator===  OutDataTypeStr=boolean  RndMeth=Simplest  InputSameDT=off
  NOT1 : Logic  Operator=NOT  IconShape=distinctive  AllPortsSameDT=off  OutDataTypeStr=boolean
  Subsystem : Subsystem
  Subsystem1 : Subsystem
  Unit Delay : UnitDelay  SampleTime=-1  HasFrameUpgradeWarning=on
  Unit Delay1 : UnitDelay  SampleTime=-1  HasFrameUpgradeWarning=on
  Close : Outport
  wires:
  In1/1 -> Demux/1
  Unit Delay1/1 -> Equal/1
  10 counts/1 -> Equal/2
  Subsystem/1(Out3) -> Unit Delay1/1
  Detect Decrease/1 -> Subsystem1/Enable
  start/1 -> Unit Delay/1
  Equal/1 -> NOT1/1
  NOT1/1 -> AND/2
  AND/1 -> Subsystem/Enable, Detect Decrease/1
  Subsystem1/1(y) -> Close/1
  Demux/1 -> Subsystem1/1(In1)
  Demux/2 -> Subsystem1/2(In2)
  Unit Delay/1 -> AND/1

== system soc_pmsm_singlecpu_ref/Current Control/ADC MidPoint Calibration/Subsystem1/If Action Subsystem ==
  In1 : Inport
  Action Port : ActionPort  ActionPortLabel=if(u1 > 1700 & u1 < 2600)
  Data Store Write1 : DataStoreWrite  DataStoreName=IaOffset  IndexOptions=Index vector (dialog)  Indices=1  OutputSizes=1
  wires:
  In1/1 -> Data Store Write1/1

== system soc_pmsm_singlecpu_ref/Current Control/ADC MidPoint Calibration/Subsystem1/If Action Subsystem1 ==
  Action Port : ActionPort  ActionPortLabel=else
  Constant : Constant  Value=inverter.CtSensAOffset  OutDataTypeStr=Inherit: Inherit via back propagation
  Data Store Write1 : DataStoreWrite  DataStoreName=IaOffset  IndexOptions=Index vector (dialog)  Indices=1  OutputSizes=1
  wires:
  Constant/1 -> Data Store Write1/1

== system soc_pmsm_singlecpu_ref/Current Control/ADC MidPoint Calibration/Subsystem1/If Action Subsystem2 ==
  In1 : Inport
  Action Port : ActionPort  ActionPortLabel=if(u1 > 1700 & u1 < 2600)
  Data Store Write2 : DataStoreWrite  DataStoreName=IbOffset  IndexOptions=Index vector (dialog)  Indices=1  OutputSizes=1
  wires:
  In1/1 -> Data Store Write2/1

== system soc_pmsm_singlecpu_ref/Current Control/ADC MidPoint Calibration/Subsystem1/If Action Subsystem3 ==
  Action Port : ActionPort  ActionPortLabel=else
  Constant1 : Constant  Value=inverter.CtSensBOffset  OutDataTypeStr=Inherit: Inherit via back propagation
  Data Store Write2 : DataStoreWrite  DataStoreName=IbOffset  IndexOptions=Index vector (dialog)  Indices=1  OutputSizes=1
  wires:
  Constant1/1 -> Data Store Write2/1

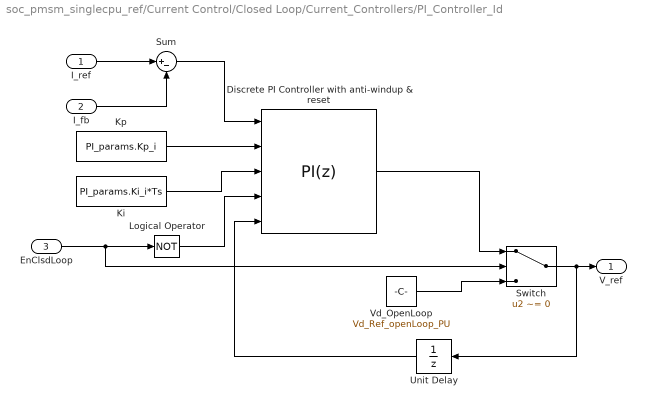
== system soc_pmsm_singlecpu_ref/Current Control/Closed Loop/Current_Controllers/PI_Controller_Id ==
  I_ref : Inport
  I_fb : Inport  Port=2
  EnClsdLoop : Inport  Port=3
  Discrete PI Controller with anti-windup & reset : slpidlib/PID Controller  Controller=PI  Form=Parallel  TimeDomain=Discrete-time  UseExternalTs=off  SampleTime=-1  IntegratorMethod=Forward Euler  FilterMethod=Forward Euler  ControllerParametersSource=external  P=1  I=1  UseKiTs=on  D=0  N=100  UseFilter=on  TunerSelectOption=Transfer Function Based (PID Tuner App)  InitialConditionSource=external  InitialConditionForIntegrator=0  InitialConditionForFilter=0  DifferentiatorICPrevScaledInput=0  ExternalReset=level  TrackingMode=off  Kt=1  LimitOutput=on  SatLimitsSource=internal  UpperSaturationLimit=1  LowerSaturationLimit=-1  LinearizeAsGain=on  AntiWindupMode=clamping  Kb=1  LimitIntegrator=off  UpperIntegratorSaturationLimit=inf  LowerIntegratorSaturationLimit=-inf  RndMeth=Simplest  POutMin=[]  POutMax=[]  IOutMin=[]  IOutMax=[]  DOutMin=[]  DOutMax=[]  NOutMin=[]  NOutMax=[]  SumOutMin=[]  SumOutMax=[]  SaturationOutDataTypeStr=Inherit: Inherit via back propagation  SaturationOutMin=[]  SaturationOutMax=[]  PParamMin=[]  PParamMax=[]  IParamMin=[]  IParamMax=[]  DParamMin=[]  DParamMax=[]  NParamMin=[]  NParamMax=[]  KbParamMin=[]  KbParamMax=[]  KtParamMin=[]  KtParamMax=[]  KbOutMin=[]  KbOutMax=[]  KtOutMin=[]  KtOutMax=[]  IntegratorOutMin=[]  IntegratorOutMax=[]  FilterOutMin=[]  FilterOutMax=[]  SumI1OutMin=[]  SumI1OutMax=[]  SumI2OutMin=[]  SumI2OutMax=[]  SumI3OutMin=[]  SumI3OutMax=[]  SumI4OutMin=[]  SumI4OutMax=[]  SumDOutMin=[]  SumDOutMax=[]  DifferentiatorOutMin=[]  DifferentiatorOutMax=[]  FilterDiffOutCoefMin=[]  FilterDiffOutCoefMax=[]  ReciprocalOutMin=[]  ReciprocalOutMax=[]  SumDenOutMin=[]  SumDenOutMax=[]  SumNumOutMin=[]  SumNumOutMax=[]  DivideOutMin=[]  DivideOutMax=[]  UdiffTsProdOutMin=[]  UdiffTsProdOutMax=[]  NTsProdOutMin=[]  NTsProdOutMax=[]  UintegralTsProdOutMin=[]  UintegralTsProdOutMax=[]  UngainTsProdOutMin=[]  UngainTsProdOutMax=[]  ClampingZeroOutDataTypeStr=Inherit: Inherit via back propagation  ClampingZeroOutMin=[]  ClampingZeroOutMax=[]  FilterDenConstantOutDataTypeStr=Inherit: Inherit via back propagation  FilterDenConstantOutMin=[]  FilterDenConstantOutMax=[]  PCopyOutDataTypeStr=Inherit: Inherit via back propagation  PCopyOutMin=[]  PCopyOutMax=[]  NCopyOutDataTypeStr=Inherit: Inherit via back propagation  NCopyOutMin=[]  NCopyOutMax=[]  IntegratorContinuousStateAttributes=''  IntegratorStateMustResolveToSignalObject=off  IntegratorRTWStateStorageClass=Auto  FilterContinuousStateAttributes=''  FilterStateMustResolveToSignalObject=off  FilterRTWStateStorageClass=Auto  ParallelPVariant=ExternalParameters  IdealPVariant=Disabled  IVariant=ExternalParameters  DVariant=Disabled  IntegratorVariant=Discrete  SatVariant=Enabled  AWVariant=DiscClampingParallel  PCopyVariant=Disabled  TRVariant=Disabled  FdbkBlocksVariant=Forward  IdealPFdbkVariant=Disabled  SatFdbkVariant=Disabled  DerivativeFilterVariant=Disabled  NVariant=Disabled  NCopyVariant=Disabled_SignalSpec  FilterICVariant=Disabled  IntegratorICVariant=ExternalICs  ExternalResetVariant=ExternalReset  TRSumVariant=Passthrough  SumFdbkVariant=Disabled  SumVariant=Sum_PI  TsampFilterVariant=InternalTs  TsampNgainVariant=Passthrough  TsampIntegralVariant=Disabled_SignalSpec  ExternalSaturationOutDataTypeStr=Inherit: Same as second input
      settings: LibrarySourceBlock=mcbcontrolslib/PI Controller
  Ki : Constant  Value=PI_params.Ki_i*Ts  OutDataTypeStr=dataType  SampleTime=-1
  Kp : Constant  Value=PI_params.Kp_i  OutDataTypeStr=dataType  SampleTime=-1
  Logical Operator : Logic  Operator=NOT  IconShape=distinctive  AllPortsSameDT=off  OutDataTypeStr=boolean
  Sum : Sum  Inputs=|+-  OutDataTypeStr=Inherit: Same as first input
  Switch : Switch  Criteria=u2 ~= 0  RndMeth=Simplest  SaturateOnIntegerOverflow=off  InputSameDT=off
  Unit Delay : UnitDelay  SampleTime=-1  HasFrameUpgradeWarning=on
  Vd_OpenLoop : Constant  Value=Vd_Ref_openLoop_PU  OutDataTypeStr=dataType  SampleTime=-1
  V_ref : Outport  VectorParamsAs1DForOutWhenUnconnected=off
  wires:
  Switch/1 -> V_ref/1, Unit Delay/1
  I_fb/1 -> Sum/2
  Sum/1 -> Discrete PI Controller with anti-windup & reset/1
  Kp/1 -> Discrete PI Controller with anti-windup & reset/2
  I_ref/1 -> Sum/1
  Ki/1 -> Discrete PI Controller with anti-windup & reset/3
  Logical Operator/1 -> Discrete PI Controller with anti-windup & reset/4
  Unit Delay/1 -> Discrete PI Controller with anti-windup & reset/5
  Discrete PI Controller with anti-windup & reset/1 -> Switch/1
  Vd_OpenLoop/1 -> Switch/3
  EnClsdLoop/1 -> Logical Operator/1, Switch/2

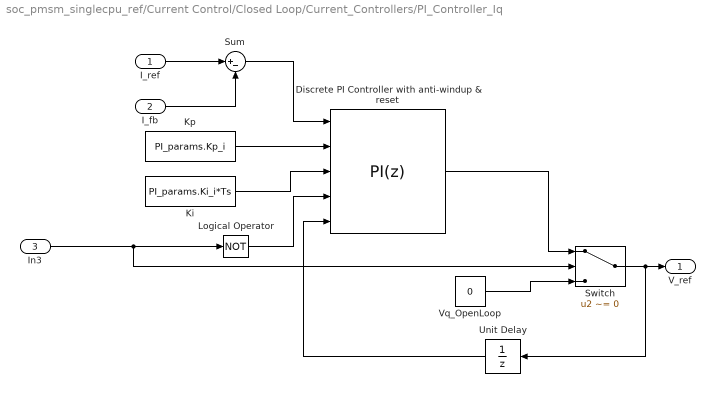
== system soc_pmsm_singlecpu_ref/Current Control/Closed Loop/Current_Controllers/PI_Controller_Iq ==
  I_ref : Inport
  I_fb : Inport  Port=2
  In3 : Inport  Port=3
  Discrete PI Controller with anti-windup & reset : slpidlib/PID Controller  Controller=PI  Form=Parallel  TimeDomain=Discrete-time  UseExternalTs=off  SampleTime=-1  IntegratorMethod=Forward Euler  FilterMethod=Forward Euler  ControllerParametersSource=external  P=1  I=1  UseKiTs=on  D=0  N=100  UseFilter=on  TunerSelectOption=Transfer Function Based (PID Tuner App)  InitialConditionSource=external  InitialConditionForIntegrator=0  InitialConditionForFilter=0  DifferentiatorICPrevScaledInput=0  ExternalReset=level  TrackingMode=off  Kt=1  LimitOutput=on  SatLimitsSource=internal  UpperSaturationLimit=1  LowerSaturationLimit=-1  LinearizeAsGain=on  AntiWindupMode=clamping  Kb=1  LimitIntegrator=off  UpperIntegratorSaturationLimit=inf  LowerIntegratorSaturationLimit=-inf  RndMeth=Simplest  POutMin=[]  POutMax=[]  IOutMin=[]  IOutMax=[]  DOutMin=[]  DOutMax=[]  NOutMin=[]  NOutMax=[]  SumOutMin=[]  SumOutMax=[]  SaturationOutDataTypeStr=Inherit: Inherit via back propagation  SaturationOutMin=[]  SaturationOutMax=[]  PParamMin=[]  PParamMax=[]  IParamMin=[]  IParamMax=[]  DParamMin=[]  DParamMax=[]  NParamMin=[]  NParamMax=[]  KbParamMin=[]  KbParamMax=[]  KtParamMin=[]  KtParamMax=[]  KbOutMin=[]  KbOutMax=[]  KtOutMin=[]  KtOutMax=[]  IntegratorOutMin=[]  IntegratorOutMax=[]  FilterOutMin=[]  FilterOutMax=[]  SumI1OutMin=[]  SumI1OutMax=[]  SumI2OutMin=[]  SumI2OutMax=[]  SumI3OutMin=[]  SumI3OutMax=[]  SumI4OutMin=[]  SumI4OutMax=[]  SumDOutMin=[]  SumDOutMax=[]  DifferentiatorOutMin=[]  DifferentiatorOutMax=[]  FilterDiffOutCoefMin=[]  FilterDiffOutCoefMax=[]  ReciprocalOutMin=[]  ReciprocalOutMax=[]  SumDenOutMin=[]  SumDenOutMax=[]  SumNumOutMin=[]  SumNumOutMax=[]  DivideOutMin=[]  DivideOutMax=[]  UdiffTsProdOutMin=[]  UdiffTsProdOutMax=[]  NTsProdOutMin=[]  NTsProdOutMax=[]  UintegralTsProdOutMin=[]  UintegralTsProdOutMax=[]  UngainTsProdOutMin=[]  UngainTsProdOutMax=[]  ClampingZeroOutDataTypeStr=Inherit: Inherit via back propagation  ClampingZeroOutMin=[]  ClampingZeroOutMax=[]  FilterDenConstantOutDataTypeStr=Inherit: Inherit via back propagation  FilterDenConstantOutMin=[]  FilterDenConstantOutMax=[]  PCopyOutDataTypeStr=Inherit: Inherit via back propagation  PCopyOutMin=[]  PCopyOutMax=[]  NCopyOutDataTypeStr=Inherit: Inherit via back propagation  NCopyOutMin=[]  NCopyOutMax=[]  IntegratorContinuousStateAttributes=''  IntegratorStateMustResolveToSignalObject=off  IntegratorRTWStateStorageClass=Auto  FilterContinuousStateAttributes=''  FilterStateMustResolveToSignalObject=off  FilterRTWStateStorageClass=Auto  ParallelPVariant=ExternalParameters  IdealPVariant=Disabled  IVariant=ExternalParameters  DVariant=Disabled  IntegratorVariant=Discrete  SatVariant=Enabled  AWVariant=DiscClampingParallel  PCopyVariant=Disabled  TRVariant=Disabled  FdbkBlocksVariant=Forward  IdealPFdbkVariant=Disabled  SatFdbkVariant=Disabled  DerivativeFilterVariant=Disabled  NVariant=Disabled  NCopyVariant=Disabled_SignalSpec  FilterICVariant=Disabled  IntegratorICVariant=ExternalICs  ExternalResetVariant=ExternalReset  TRSumVariant=Passthrough  SumFdbkVariant=Disabled  SumVariant=Sum_PI  TsampFilterVariant=InternalTs  TsampNgainVariant=Passthrough  TsampIntegralVariant=Disabled_SignalSpec  ExternalSaturationOutDataTypeStr=Inherit: Same as second input
      settings: LibrarySourceBlock=mcbcontrolslib/PI Controller
  Ki : Constant  Value=PI_params.Ki_i*Ts  OutDataTypeStr=dataType  SampleTime=-1
  Kp : Constant  Value=PI_params.Kp_i  OutDataTypeStr=dataType  SampleTime=-1
  Logical Operator : Logic  Operator=NOT  IconShape=distinctive  AllPortsSameDT=off  OutDataTypeStr=boolean
  Sum : Sum  Inputs=|+-  OutDataTypeStr=Inherit: Same as first input
  Switch : Switch  Criteria=u2 ~= 0  RndMeth=Simplest  SaturateOnIntegerOverflow=off  InputSameDT=off
  Unit Delay : UnitDelay  SampleTime=-1  HasFrameUpgradeWarning=on
  Vq_OpenLoop : Constant  Value=0  OutDataTypeStr=dataType  SampleTime=-1
  V_ref : Outport  VectorParamsAs1DForOutWhenUnconnected=off
  wires:
  Switch/1 -> V_ref/1, Unit Delay/1
  I_fb/1 -> Sum/2
  Sum/1 -> Discrete PI Controller with anti-windup & reset/1
  Kp/1 -> Discrete PI Controller with anti-windup & reset/2
  I_ref/1 -> Sum/1
  Ki/1 -> Discrete PI Controller with anti-windup & reset/3
  Logical Operator/1 -> Discrete PI Controller with anti-windup & reset/4
  Unit Delay/1 -> Discrete PI Controller with anti-windup & reset/5
  Discrete PI Controller with anti-windup & reset/1 -> Switch/1
  Vq_OpenLoop/1 -> Switch/3
  In3/1 -> Logical Operator/1, Switch/2

== system soc_pmsm_singlecpu_ref/Current Control/Input Scaling/Calculate Phase Currents/Data_Type ==
  In1 : Inport
  Data_Type_Fixed_Point : Subsystem  VariantControl=~isequal(dataType,'single')
  Data_Type_Float : Subsystem  VariantControl=isequal(dataType,'single')
  Iab_meas_PU : Outport

== system soc_pmsm_singlecpu_ref/Current Control/Input Scaling/Calculate position and speed/Flux Observer ==
  note: This filter introduces pole and zero cancellation happens in speed loop
  InputSignals : Inport
  Constant : Constant  SampleTime=-1
  Demux2 : Demux
  Flux Observer : mcbpositiondecoderlib/Flux Observer  MotorSelection=PMSM  DataTypeSelect=off  BlockInputUnit=Per-unit  PerUnitVoltage=PU_System.V_base  PerUnitCurrent=PU_System.I_base  PositionSelect=on  FluxSelect=off  TorqueSelect=off  PolePairs=4  StatorResistance=pmsm.Rs  StatorDAxisInductance=pmsm.Ld  StatorLeakageInductance=0.0068  RotorLeakageInductance=0.0068  MagnetizingInductance=0.0300  CutoffFreq=3.1863  BlockSampleTime=Ts  PositionUnit=Per-unit  PositionDatatype=dataType  FluxUnit=Weber  PerUnitFlux=0.1  FluxDatatype=single  TorqueUnit=Nm  PerUnitTorque=100  TorqueDatatype=single  DataType=0
  IIR Filter4 : mcbcontrolslib/IIR Filter  VariantControl=Low Pass Filter  VariantSelect=Low-pass  Filter_constant=0.01  advancedSettings=off  Ts=50e-6  cutOff_freq=32.1525
  Logical Operator : Logic  Operator=NOT  IconShape=distinctive  AllPortsSameDT=off  OutDataTypeStr=boolean
  Mux2 : Mux  Inputs=2
  Speed Measurement : mcbpositiondecoderlib/Speed Measurement  PositionUnit=Per unit  PositionScalingDatatype=uint32  SpeedCalculationMode=Time interval for speed calculation  SampleTimeAsync=Ts  MaximumApplicationSpeed=60000  SpeedResolution=5e-6  DelayLength=10  MaximumMeasurableSpeed=59999  MeasurableSpeedResolution=2.794e-05  SpeedUnit=Per unit based on dialog  PerUnitSpeed=PU_System.N_base  SpeedDataType=dataType
  elect2mech : Gain  Gain=1/pmsm.p  RndMeth=Simplest  OutDataTypeStr=Inherit: Same as input
  Position/Speed : Outport
  wires:
  InputSignals/1 -> Demux2/1
  Demux2/1 -> Flux Observer/1
  Demux2/2 -> Flux Observer/2
  Mux2/1 -> Position/Speed/1
  Speed Measurement/1 -> IIR Filter4/1
  elect2mech/1 -> Mux2/2
  Demux2/3 -> Flux Observer/3  "Ialpha"
  Demux2/4 -> Flux Observer/4  "Ibeta"
  IIR Filter4/1 -> elect2mech/1
  Flux Observer/1 -> Mux2/1, Speed Measurement/1
  Logical Operator/1 -> Flux Observer/5
  Constant/1 -> Logical Operator/1

== system soc_pmsm_singlecpu_ref/Current Control/Open_Loop_Control/Subsystem/Subsystem ==
  Enable : EnablePort
  Counter Free-Running : simulink/Sources/Counter Free-Running  NumBits=16  tsamp=-1
  Out3 : Outport  InitialOutput=0
  wires:
  Counter Free-Running/1 -> Out3/1

== system soc_pmsm_singlecpu_ref/Current Control/Open_Loop_Control/Subsystem/Subsystem1 ==
  note: if any one has a significant differene, then currents are raising
      | Downside, if noise is more this might not work, so not enabling
  In1 : Inport
  In2 : Inport  Port=2
  Enable : EnablePort
  Abs2 : Abs  SaturateOnIntegerOverflow=off
  Constant3 : Constant  Value=50
  GreaterThan2 : RelationalOperator  Operator=>  OutDataTypeStr=boolean  RndMeth=Simplest  InputSameDT=off
  Minus : Sum  Inputs=+-
  y : Outport
  wires:
  In1/1 -> Minus/1
  In2/1 -> Minus/2
  Minus/1 -> Abs2/1
  Abs2/1 -> GreaterThan2/1
  Constant3/1 -> GreaterThan2/2
  GreaterThan2/1 -> y/1

== system soc_pmsm_singlecpu_ref/Current Control/Input Scaling/Calculate Phase Currents/Data_Type/Data_Type_Fixed_Point ==
  In1 : Inport
  Data Type Conversion : DataTypeConversion  OutDataTypeStr=fixdt(1,32,17)  ConvertRealWorld=Stored Integer (SI)  RndMeth=Simplest  SaturateOnIntegerOverflow=off
  Data Type Conversion1 : DataTypeConversion  OutDataTypeStr=dataType  RndMeth=Simplest  SaturateOnIntegerOverflow=off
  Q17 per unit conversion : ArithShift  BitShiftNumber=-6
  Iab_meas_PU : Outport
  wires:
  In1/1 -> Q17 per unit conversion/1
  Data Type Conversion1/1 -> Iab_meas_PU/1
  Data Type Conversion/1 -> Data Type Conversion1/1
  Q17 per unit conversion/1 -> Data Type Conversion/1

== system soc_pmsm_singlecpu_ref/Current Control/Input Scaling/Calculate Phase Currents/Data_Type/Data_Type_Float ==
  In1 : Inport
  Current Sense Gain : Gain  Gain=PU_System.I_base/1.65  RndMeth=Simplest  OutDataTypeStr=Inherit: Same as input
  Get_ADC_Volt : Gain  Gain=1.65/2048  OutDataTypeStr=dataType  RndMeth=Simplest
  PU_Conversion : Gain  Gain=1/PU_System.I_base  RndMeth=Simplest  OutDataTypeStr=Inherit: Same as input
  Iab_meas_PU : Outport
  wires:
  Current Sense Gain/1 -> PU_Conversion/1
  In1/1 -> Get_ADC_Volt/1
  Get_ADC_Volt/1 -> Current Sense Gain/1
  PU_Conversion/1 -> Iab_meas_PU/1
